simulink model "project7"  (R2020b)
settings: Solver=VariableStepAuto  StartTime=0.0  StopTime=10.0  RelTol=1e-3
libraries: simulink x1
settings Model: Creator=admin  LastModifiedBy=admin

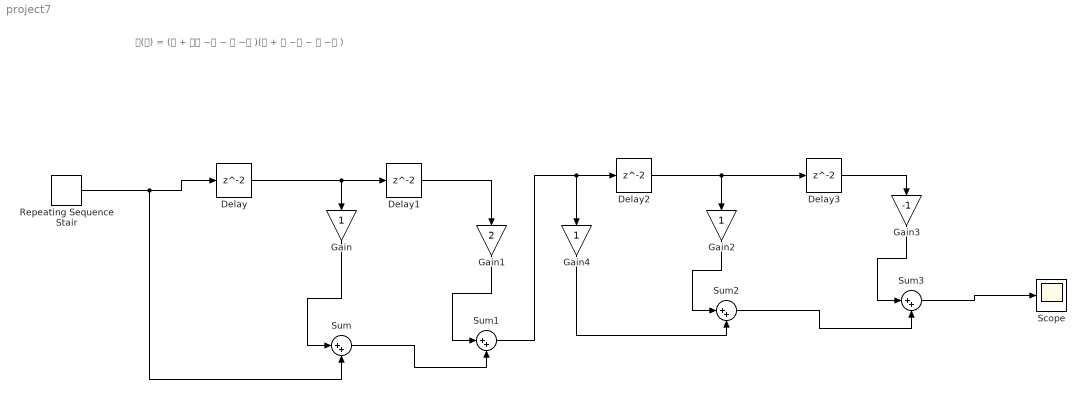
== system project7 ==
  note: 𝐇(𝐳) = (𝟏 + 𝟐𝐳 −𝟏 − 𝐳 −𝟐 )(𝟏 + 𝐳 −𝟏 − 𝐳 −𝟐 )
  Delay{,1..3} (4 alike) : Delay
  Gain : Gain
  Gain1 : Gain  Gain=2
  Gain2 : Gain
  Gain3 : Gain  Gain=-1
  Gain4 : Gain
  Repeating Sequence Stair : simulink/Sources/Repeating Sequence Stair  OutValues=[3 1 4 2 1].'  tsamp=-1  OutMin=[]  OutMax=[]  OutDataTypeStr=double  OutputDataTypeScalingMode=double  OutDataType=fixdt(0,8)  ConRadixGroup=Best Precision: Vector-wise  OutScaling=2^-12
  Scope : Scope
  Sum{,1..3} (4 alike) : Sum  Inputs=|++
  wires:
  Gain/1 -> Sum/1
  Repeating Sequence Stair/1 -> Delay/1, Sum/2
  Delay1/1 -> Gain1/1
  Delay/1 -> Gain/1, Delay1/1
  Gain1/1 -> Sum1/1
  Sum/1 -> Sum1/2
  Sum1/1 -> Delay2/1, Gain4/1
  Gain4/1 -> Sum2/2
  Gain2/1 -> Sum2/1
  Delay2/1 -> Gain2/1, Delay3/1
  Sum2/1 -> Sum3/2
  Gain3/1 -> Sum3/1
  Sum3/1 -> Scope/1
  Delay3/1 -> Gain3/1
